simulink model "task6"  (R2020b)
settings: Solver=VariableStepAuto  StartTime=0.0  StopTime=100.0  RelTol=1e-3
settings Model: Creator=zceexdu  LastModifiedBy=zceexdu

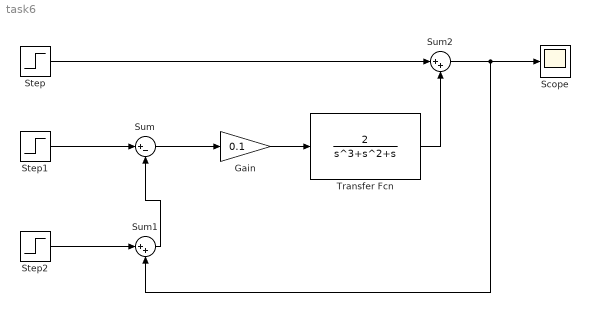
== system task6 ==
  Gain : Gain  Gain=0.1
  Scope : Scope
  Step : Step  SampleTime=0
  Step1 : Step  After=100  SampleTime=0
  Step2 : Step  SampleTime=0
  Sum : Sum  Inputs=|+-
  Sum1 : Sum  Inputs=|++
  Sum2 : Sum  Inputs=|++
  Transfer Fcn : TransferFcn  Numerator=[2]  Denominator=[1 1 1 0]
  wires:
  Step/1 -> Sum2/1
  Sum2/1 -> Sum1/2, Scope/1
  Transfer Fcn/1 -> Sum2/2
  Step1/1 -> Sum/1
  Sum/1 -> Gain/1
  Gain/1 -> Transfer Fcn/1
  Step2/1 -> Sum1/1
  Sum1/1 -> Sum/2
